simulink library "BAMLIB564xL"  (R2016b)
settings: Solver=FixedStepDiscrete  StartTime=0.0  StopTime=10.0  RelTol=1e-3  EnableMultiTasking=on
undefined symbols (not defined in the file or in its folder): Kx, Ky, ps32Table, s32A1, s32A2, s32ArgDcBusMsr, s32B0, s32B1, s32B2, s32CC1, s32CC2, s32HystOff, s32HystOn, s32IntegGain, s32LowerLim, s32LowerLimit, s32MidId, s32MidIdx, s32ModIndex, s32OutValOff, s32OutValOn, s32PropGain, s32RampDown, s32RampUp, s32ShamOffset, s32ShamOffset1, s32ShamOffset2, s32UpperLimit, ThetaAdj
undefined symbols (not defined in the file): CoefBuf, Order, s32C1, s32Kd, s32Kq, s32Lim, s32UpperLim, u16NSamples
(part 1 of 2)
settings Model: Creator=r61406  LastModifiedBy=eugkim01
settings SolverCC: PositivePriorityOrder=on  AutoInsertRateTranBlk=on
settings DataIOCC: LimitDataPoints=on  SaveFormat=Array  SignalLoggingSaveFormat=ModelDataLogs
settings OptimizationCC: ExpressionDepthLimit=2147483647  LifeSpan=1
settings DebuggingCC: UnderspecifiedInitializationDetection=Classic  MergeDetectMultiDrivingBlocksExec=none  SolverPrmCheckMsg=warning  FcnCallInpInsideContextMsg=warning  StateNameClashWarn=warning  StrictBusMsg=Warning  SFUnexpectedBacktrackingDiag=warning  SFNoUnconditionalDefaultTransitionDiag=warning  SFExecutionAtInitializationDiag=none
settings HardwareCC: ProdBitPerPointer=32  ProdBitPerSizeT=32  ProdBitPerPtrDiffT=32  ProdLargestAtomicFloat=None  ProdIntDivRoundTo=Undefined  ProdEndianess=Unspecified  ProdWordSize=32  ProdHWDeviceType=32-bit Generic
settings ModelReferenceCC: PropagateSignalLabelsOutOfModel=off
settings RTWCC: SystemTargetFile=ert.tlc  TemplateMakefile=ert_default_tmf  Description=Real-Time Workshop Embedded Coder (no auto configuration)  GenerateReport=on  IncludeHyperlinkInReport=on  LaunchReport=on  GenerateTraceInfo=on  GenerateTraceReport=on  GenerateTraceReportSl=on  GenerateTraceReportSf=on  GenerateTraceReportEml=on
settings CodeAppCC: IgnoreCustomStorageClasses=off  CustomSymbolStrType=$N$R$M  InternalIdentifier=Classic
settings ERTTargetCC: GenerateSampleERTMain=on  ERTCustomFileTemplate=example_file_process.tlc  ConvertIfToSwitch=off  SuppressUnreachableDefaultCases=off
settings ConfigComp: CovMetricSettings=dw  CovHtmlReporting=on  CovSaveCumulativeToWorkspaceVar=on  CovSaveSingleToWorkspaceVar=on  CovExternalEMLEnable=off

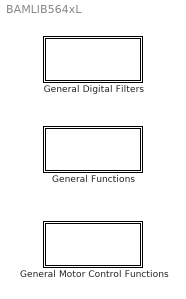
== system BAMLIB564xL ==
  General Digital Filters : Subsystem
      mask Display: disp('GDFLIB')
  General Functions : Subsystem
      mask Display: disp('GFLIB')
  General Motor Control Functions : Subsystem
      mask Display: disp('GMCLIB')

== system BAMLIB564xL/General Digital Filters ==
  GDFLIB_FilterFIR : Subsystem  mask(GDFLIB_FilterFIR){u32Order=Order, ps32CoefBuf=CoefBuf}
      mask help: The function implements FIR filter.
      mask init:
      | pos = get_param(gcb, 'Position');width = pos(3) - pos(1); height = pos(4) - pos(2);tX=width/2;tY=height*0.9;
      mask Help: web([rappid_564xl_mc_block_help,filesep,'help.html']);
      mask Display:
      | color('black');port_label('input',1,'singleIn');port_label('output',1,'singleOut');color('black');disp('GDFLIB_FilterFIR');
      | color('blue');
      | text(tX,tY, 'BAM', 'horizontalalignment', 'center');
  GDFLIB_FilterIIR1 : Subsystem  mask(GDFLIB_FilterIIR1){s32B0=s32B0, s32B1=s32B1, s32A1=s32A1}
      mask help: Bit accurate model of first order IIR filter. All parameters as well as input and output are integers.
      mask init:
      | pos = get_param(gcb, 'Position');width = pos(3) - pos(1); height = pos(4) - pos(2);tX=width/2;tY=height*0.9;
      mask Help: web([rappid_564xl_mc_block_help,filesep,'help.html']);
      mask Display: color('black');port_label('input',1,'singleIn');port_label('output',1,'singleOut');color('black');disp('GDFLIB_FilterIIR1');color('blue');text(tX,tY, 'BAM', 'horizontalAlignment', 'center');
  GDFLIB_FilterIIR2 : Subsystem  mask(GDFLIB_FilterIIR2){s32B0=s32B0, s32B1=s32B1, s32B2=s32B2, s32A1=s32A1, s32A2=s32A2}
      mask help: Bit accurate model of direct form I second order IIR filter. All parameters as well as input and output are integers.
      mask init:
      | pos = get_param(gcb, 'Position');width = pos(3) - pos(1); height = pos(4) - pos(2);tX=width/2;tY=height*0.9;
      mask Help: web([rappid_564xl_mc_block_help,filesep,'help.html']);
      mask Display: color('black');port_label('input',1,'singleIn');port_label('output',1,'singleOut');color('black');disp('GDFLIB_FilterIIR2');color('blue');text(tX,tY, 'BAM', 'horizontalAlignment', 'center');
  GDFLIB_FilterMA : Subsystem  mask(GDFLIB_FilterMA){u16NSamples=u16NSamples}
      mask help: Bit accurate model of recursive form moving average filter. All parameters as well as input and output are 32bit integers.
      mask init:
      | pos = get_param(gcb, 'Position');width = pos(3) - pos(1); height = pos(4) - pos(2);tX=width/2;tY=height*0.9;
      mask Help: web([rappid_564xl_mc_block_help,filesep,'help.html']);
      mask Display: color('black');port_label('input',1,'singleIn');port_label('output',1,'singleOut');color('black');disp('GDFLIB_FilterMA');color('blue');text(tX,tY, 'BAM', 'horizontalAlignment', 'center');

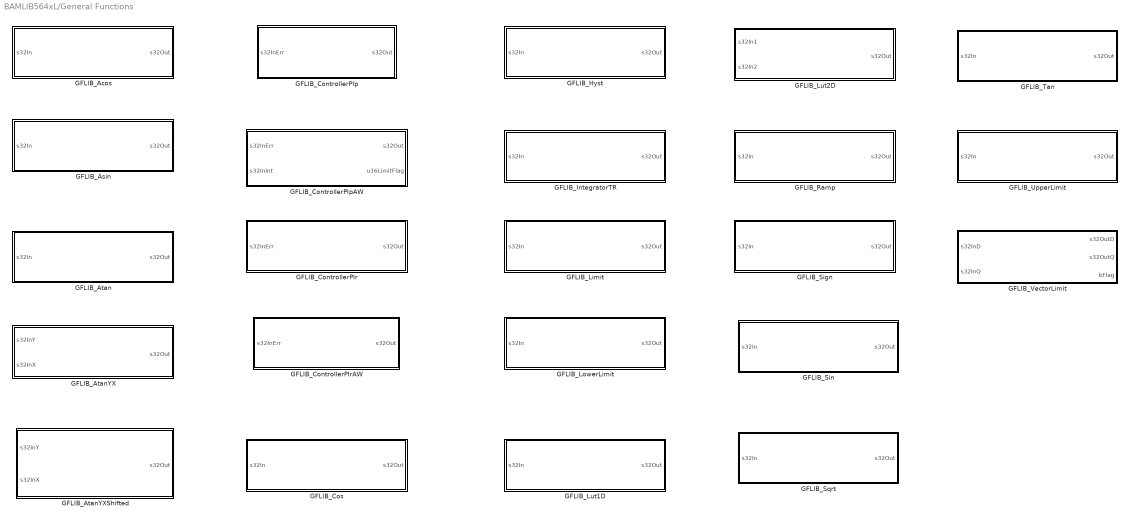
== system BAMLIB564xL/General Functions ==
  GFLIB_Acos : Subsystem  mask(GFLIB_Acos){}
      mask help: Bit accurate model of GFLIB_Acos function, which computes the acos(single) using the 4th order Taylor polynomial approximation.
      mask init:
      | pos = get_param(gcb, 'Position');width = pos(3) - pos(1); height = pos(4) - pos(2);tX=width/2;tY=height*0.9;
      mask Help: web([rappid_564xl_mc_block_help,filesep,'help.html']);
      mask Display: color('black');port_label('input',1,'singleIn');port_label('output',1,'singleOut');color('black');disp('GFLIB_Acos');color('blue');text(tX,tY, 'BAM', 'horizontalAlignment', 'center');
  GFLIB_Asin : Subsystem  mask(GFLIB_Asin){}
      mask help: Bit accurate model of GFLIB_Asin function, which computes the asin(single) using the 4th order Taylor polynomial approximation.
      mask init:
      | pos = get_param(gcb, 'Position');width = pos(3) - pos(1); height = pos(4) - pos(2);tX=width/2;tY=height*0.9;
      mask Help: web([rappid_564xl_mc_block_help,filesep,'help.html']);
      mask Display: color('black');port_label('input',1,'singleIn');port_label('output',1,'singleOut');color('black');disp('GFLIB_Asin');color('blue');text(tX,tY, 'BAM', 'horizontalAlignment', 'center');
  GFLIB_Atan : Subsystem  mask(GFLIB_Atan){}
      mask help: Bit accurate model of GFLIB_Atan function, which computes the atan(single) using the 4th order Taylor polynomial approximation.
      mask init:
      | pos = get_param(gcb, 'Position');width = pos(3) - pos(1); height = pos(4) - pos(2);tX=width/2;tY=height*0.9;
      mask Help: web([rappid_564xl_mc_block_help,filesep,'help.html']);
      mask Display: color('black');port_label('input',1,'singleIn');port_label('output',1,'singleOut');color('black');disp('GFLIB_Atan');color('blue');text(tX,tY, 'BAM', 'horizontalAlignment', 'center');
  GFLIB_AtanYX : Subsystem  mask(GFLIB_AtanYX){}
      mask help: Bit accurate model of GFLIB_AtanYX function.
      mask init:
      | pos = get_param(gcb, 'Position');width = pos(3) - pos(1); height = pos(4) - pos(2);tX=width/2;tY=height*0.9;
      mask Help: web([rappid_564xl_mc_block_help,filesep,'help.html']);
      mask Display: color('black');port_label('input',1,'singleInY');port_label('input',2,'singleInX');port_label('output',1,'singleOut');color('black');disp('GFLIB_AtanYX');color('blue');text(tX,tY, 'BAM', 'horizontalAlignment', 'center');
  GFLIB_AtanYXShifted : Subsystem  mask{Ky=Ky, Kx=Kx, ThetaAdj=ThetaAdj}
      mask help: Bit accurate model of AtanYXShifted function
      mask init:
      | pos = get_param(gcb, 'Position');width = pos(3) - pos(1); height = pos(4) - pos(2);tX=width/2;tY=height*0.9;
      mask Help: web([rappid_564xl_mc_block_help,filesep,'help.html']);
      mask Display:
      | color('black');
      | port_label('input',1, 'singleInY');
      | port_label('input',2, 'singleInX');
      | port_label('output', 1, 'singleOut');
      | color('black');
      | disp('GFLIB_AtanYXShifted');
      | color('blue');
      | text(tX,tY, 'BAM', 'horizontalAlignment', 'center');
  GFLIB_ControllerPIp : Subsystem  mask(GFLIB_ControllerPIp){s32PropGain=s32PropGain, s32IntegGain=s32IntegGain}
      mask help: Bit accurate model of parallel form PI controller without anti-windup. All parameters as well as input and output are integers.
      mask init:
      | pos = get_param(gcb, 'Position');width = pos(3) - pos(1); height = pos(4) - pos(2);tX=width/2;tY=height*0.9;
      mask Help: web([rappid_564xl_mc_block_help,filesep,'help.html']);
      mask Display: color('black');port_label('input',1,'singleInErr');port_label('output',1,'singleOut');color('black');disp('GFLIB_ControllerPIp');color('blue');text(tX,tY, 'BAM', 'horizontalAlignment', 'center');
  GFLIB_ControllerPIpAW : Subsystem  mask(GFLIB_ControllerPIpAW){s32PropGain=s32PropGain, s32IntegGain=s32IntegGain, s32UpperLimit=s32UpperLimit, s32LowerLimit=s32LowerLimit}
      mask help: Bit accurate model of parallel form PI controller with anti-windup. All parameters as well as input and output are single precision float.
      mask init:
      | pos = get_param(gcb, 'Position');width = pos(3) - pos(1); height = pos(4) - pos(2);tX=width/2;tY=height*0.9;
      mask Help: web([rappid_564xl_mc_block_help,filesep,'help.html']);
      mask Display: color('black');port_label('input',1,'singleInErr');port_label('output',1,'singleOut');port_label('output',2,'u16LimitFlag');color('black');disp('GFLIB_ControllerPIpAW');color('blue');text(tX,tY, 'BAM', 'horizontalAlignment', 'center');
  GFLIB_ControllerPIr : Subsystem  mask(GFLIB_ControllerPIr){s32CC1=s32CC1, s32CC2=s32CC2}
      mask help: Bit accurate model of reccurent form Pi controller without anti-windup. All parameters as well as input and output are single precision floating point.
      mask init:
      | pos = get_param(gcb, 'Position');width = pos(3) - pos(1); height = pos(4) - pos(2);tX=width/2;tY=height*0.9;
      mask Help: web([rappid_564xl_mc_block_help,filesep,'help.html']);
      mask Display: color('black');port_label('input',1,'singleInErr');port_label('output',1,'singleOut');color('black');disp('GFLIB_ControllerPIr');color('blue');text(tX,tY, 'BAM', 'horizontalAlignment', 'center');
  GFLIB_ControllerPIrAW : Subsystem  mask(GFLIB_ControllerPIrAW){s32CC1=s32CC1, s32CC2=s32CC2, s32UpperLimit=s32UpperLimit, s32LowerLimit=s32LowerLimit}
      mask help: Bit accurate model of reccurent form PI controller with anti-windup. All parameters as well as input and output are 32bit integers except for u16NShift parameter which is 16bit unsigned integer.
      mask init:
      | pos = get_param(gcb, 'Position');width = pos(3) - pos(1); height = pos(4) - pos(2);tX=width/2;tY=height*0.9;
      mask Help: web([rappid_564xl_mc_block_help,filesep,'help.html']);
      mask Display: color('black');port_label('input',1,'singleInErr');port_label('output',1,'singleOut');color('black');disp('GFLIB_ControllerPIrAW');color('blue');text(tX,tY, 'BAM', 'horizontalAlignment', 'center');
  GFLIB_Cos : Subsystem  mask(GFLIB_Cos){}
      mask help: Bit accurate model of GFLIB_Cos function, which computes the cos(pi * single) using the 9th order Taylor polynomial approximation.
      mask init:
      | pos = get_param(gcb, 'Position');width = pos(3) - pos(1); height = pos(4) - pos(2);tX=width/2;tY=height*0.9;
      mask Help: web([rappid_564xl_mc_block_help,filesep,'help.html']);
      mask Display: color('black');port_label('input',1,'singleIn');port_label('output',1,'singleOut');color('black');disp('GFLIB_Cos');color('blue');text(tX,tY, 'BAM', 'horizontalAlignment', 'center');
  GFLIB_Hyst : Subsystem  mask(GFLIB_Hyst){s32HystOn=s32HystOn, s32HystOff=s32HystOff, s32OutValOn=s32OutValOn, s32OutValOff=s32OutValOff}
      mask help: Bit accurate model of hysteresis function. All parameters as well as input and output are 32bit integers.
      mask init:
      | pos = get_param(gcb, 'Position');width = pos(3) - pos(1); height = pos(4) - pos(2);tX=width/2;tY=height*0.9;
      mask Help: web([rappid_564xl_mc_block_help,filesep,'help.html']);
      mask Display: color('black');port_label('input',1,'singleIn');port_label('output',1,'singleOut');color('black');disp('GFLIB_Hyst');color('blue');text(tX,tY, 'BAM', 'horizontalAlignment', 'center');
  GFLIB_IntegratorTR : Subsystem  mask(GFLIB_IntegratorTR){s32C1=s32C1}
      mask help: Bit accurate model of discrete trapezoidal integrator. All parameters as well as input and output are 32bit integers.
      mask init:
      | pos = get_param(gcb, 'Position');width = pos(3) - pos(1); height = pos(4) - pos(2);tX=width/2;tY=height*0.9;
      mask Help: web([rappid_564xl_mc_block_help,filesep,'help.html']);
      mask Display: color('black');port_label('input',1,'singleIn');port_label('output',1,'singleOut');color('black');disp('GFLIB_IntegratorTR');color('blue');text(tX,tY, 'BAM', 'horizontalAlignment', 'center');
  GFLIB_Limit : Subsystem  mask(GFLIB_Limit){s32UpperLimit=s32UpperLimit, s32LowerLim=s32LowerLim}
      mask help: Bit accurate model of GFLIB_Limit function
      mask init:
      | pos = get_param(gcb, 'Position');width = pos(3) - pos(1); height = pos(4) - pos(2);tX=width/2;tY=height*0.9;
      mask Help: web([rappid_564xl_mc_block_help,filesep,'help.html']);
      mask Display: color('black');port_label('input',1,'singleIn');port_label('output',1,'singleOut');color('black');disp('GFLIB_Limit');color('blue');text(tX,tY, 'BAM', 'horizontalAlignment', 'center');
  GFLIB_LowerLimit : Subsystem  mask(GFLIB_LowerLimit){s32LowerLim=s32LowerLim}
      mask help: Bit accurate model of GFLIB_LowerLimit function
      mask init:
      | pos = get_param(gcb, 'Position');width = pos(3) - pos(1); height = pos(4) - pos(2);tX=width/2;tY=height*0.9;
      mask Help: web([rappid_564xl_mc_block_help,filesep,'help.html']);
      mask Display: color('black');port_label('input',1,'singleIn');port_label('output',1,'singleOut');color('black');disp('GFLIB_LowerLimit');color('blue');text(tX,tY, 'BAM', 'horizontalAlignment', 'center');
  GFLIB_Lut1D : Subsystem  mask(GFLIB_Lut1D){s32ShamOffset=s32ShamOffset, ps32Table=ps32Table, s32MidIdx=s32MidIdx}
      mask help: Bit accurate model of GFLIB_Lut1D function
      mask init:
      | pos = get_param(gcb, 'Position');width = pos(3) - pos(1); height = pos(4) - pos(2);tX=width/2;tY=height*0.9;
      mask Help: web([rappid_564xl_mc_block_help,filesep,'help.html']);
      mask Display: color('black');port_label('input',1,'singleIn');port_label('output',1,'singleOut');color('black');disp('GFLIB_Lut1D');color('blue');text(tX,tY, 'BAM', 'horizontalAlignment', 'center');
  GFLIB_Lut2D : Subsystem  mask(GFLIB_Lut2D){s32ShamOffset1=s32ShamOffset1, s32ShamOffset2=s32ShamOffset2, ps32Table=ps32Table, s32MidId=s32MidId}
      mask help: Bit accurate model of GFLIB_Lut2D function
      mask init:
      | pos = get_param(gcb, 'Position');width = pos(3) - pos(1); height = pos(4) - pos(2);tX=width/2;tY=height*0.9;
      mask Help: web([rappid_564xl_mc_block_help,filesep,'help.html']);
      mask Display: color('black');port_label('input',1,'singleIn1');port_label('input',2,'singleIn2');port_label('output',1,'singleOut');color('black');disp('GFLIB_Lut2D');color('blue');text(tX,tY, 'BAM', 'horizontalAlignment', 'center');
  GFLIB_Ramp : Subsystem  mask(GFLIB_Ramp){s32RampUp=s32RampUp, s32RampDown=s32RampDown}
      mask help: Bit accurate model of ramp function. All parameters as well as input and output are 32bit integers.
      mask init:
      | pos = get_param(gcb, 'Position');width = pos(3) - pos(1); height = pos(4) - pos(2);tX=width/2;tY=height*0.9;
      mask Help: web([rappid_564xl_mc_block_help,filesep,'help.html']);
      mask Display: color('black');port_label('input',1,'singleIn');port_label('output',1,'singleOut');color('black');disp('GFLIB_Ramp');color('blue');text(tX,tY, 'BAM', 'horizontalAlignment', 'center');
  GFLIB_Sign : Subsystem  mask(GFLIB_Sign){}
      mask help: Bit accurate model of Sign function
      mask init:
      | pos = get_param(gcb, 'Position');width = pos(3) - pos(1); height = pos(4) - pos(2);tX=width/2;tY=height*0.9;
      mask Help: web([rappid_564xl_mc_block_help,filesep,'help.html']);
      mask Display: color('black');port_label('input',1,'singleIn');port_label('output',1,'singleOut');color('black');disp('GFLIB_Sign');color('blue');text(tX,tY, 'BAM', 'horizontalAlignment', 'center');
  GFLIB_Sin : Subsystem  mask(GFLIB_Sin){}
      mask help: Bit accurate model of GFLIB_Sin function, which computes the sin(pi * single) using the 9th order Taylor polynomial approximation.
      mask init:
      | pos = get_param(gcb, 'Position');width = pos(3) - pos(1); height = pos(4) - pos(2);tX=width/2;tY=height*0.9;
      mask Help: web([rappid_564xl_mc_block_help,filesep,'help.html']);
      mask Display: color('black');port_label('input',1,'singleIn');port_label('output',1,'singleOut');color('black');disp('GFLIB_Sin');color('blue');text(tX,tY, 'BAM', 'horizontalAlignment', 'center');
  GFLIB_Sqrt : Subsystem  mask(GFLIB_Sqrt){}
      mask help: Bit accurate model of GFLIB_Sqrt function, which computes the square root of input argument using the Newton-Raphson iterations preceeded by normalization and tentative approximation.
      mask init:
      | pos = get_param(gcb, 'Position');width = pos(3) - pos(1); height = pos(4) - pos(2);tX=width/2;tY=height*0.9;
      mask Help: web([rappid_564xl_mc_block_help,filesep,'help.html']);
      mask Display: color('black');port_label('input',1,'singleIn');port_label('output',1,'singleOut');color('black');disp('GFLIB_Sqrt');color('blue');text(tX,tY, 'BAM', 'horizontalAlignment', 'center');
  GFLIB_Tan : Subsystem  mask(GFLIB_Tan){}
      mask help: Bit accurate model of GFLIB_Tan function, which computes the tan(pi * single) using the 4th order Taylor polynomial approximation.
      mask init:
      | pos = get_param(gcb, 'Position');width = pos(3) - pos(1); height = pos(4) - pos(2);tX=width/2;tY=height*0.9;
      mask Help: web([rappid_564xl_mc_block_help,filesep,'help.html']);
      mask Display: color('black');port_label('input',1,'singleIn');port_label('output',1,'singleOut');color('black');disp('GFLIB_Tan');color('blue');text(tX,tY, 'BAM', 'horizontalAlignment', 'center');
  GFLIB_UpperLimit : Subsystem  mask(GFLIB_UpperLimit){s32UpperLim=s32UpperLim}
      mask help: Bit accurate model of GFLIB_UpperLimit function
      mask init:
      | pos = get_param(gcb, 'Position');width = pos(3) - pos(1); height = pos(4) - pos(2);tX=width/2;tY=height*0.9;
      mask Help: web([rappid_564xl_mc_block_help,filesep,'help.html']);
      mask Display: color('black');port_label('input',1,'singleIn');port_label('output',1,'singleOut');color('black');disp('GFLIB_UpperLimit');color('blue');text(tX,tY, 'BAM', 'horizontalAlignment', 'center');
  GFLIB_VectorLimit : Subsystem  mask(GFLIB_VectorLimit){s32Lim=s32Lim}
      mask help: Bit accurate model of GFLIB_VectorLimit function
      mask init:
      | pos = get_param(gcb, 'Position');width = pos(3) - pos(1); height = pos(4) - pos(2);tX=width/2;tY=height*0.9;
      mask Help: web([rappid_564xl_mc_block_help,filesep,'help.html']);
      mask Display: color('black');port_label('input',1,'singleInD');port_label('input',2,'singleInQ');port_label('output',1,'singleOutD');port_label('output',2,'singleOutQ');port_label('output',3,'bFlag');color('black');disp('GFLIB_VectorLimit');color('blue');text(tX,tY, 'BAM', 'horizontalAlignment', 'center');

== system BAMLIB564xL/General Motor Control Functions ==
  GMCLIB_Clark : Subsystem  mask(GMCLIB_Clark){}
      mask help: Bit accurate model of Clarke transformation 3ph -> 2ph
      mask init:
      | pos = get_param(gcb, 'Position');width = pos(3) - pos(1); height = pos(4) - pos(2);tX=width/2;tY=height*0.9;
      mask Help: web([rappid_564xl_mc_block_help,filesep,'help.html']);
      mask Display: color('black');port_label('input',1,'singleA');port_label('input',2,'singleB');port_label('input',3,'singleC');port_label('output',1,'singleAlpha');port_label('output',2,'singleBeta');color('black');disp('GMCLIB_Clark');color('blue');text(tX,tY, 'BAM', 'horizontalAlignment', 'center');
  GMCLIB_ClarkInv : Subsystem  mask(GMCLIB_ClarkInv){}
      mask help: Bit accurate model of inverse Clarke transformation 2ph -> 3ph
      mask init:
      | pos = get_param(gcb, 'Position');width = pos(3) - pos(1); height = pos(4) - pos(2);tX=width/2;tY=height*0.9;
      mask Help: web([rappid_564xl_mc_block_help,filesep,'help.html']);
      mask Display: color('black');port_label('input',1,'singleAlpha');port_label('input',2,'singleBeta');port_label('output',1,'singleA');port_label('output',2,'singleB');port_label('output',3,'singleC');color('black');disp('GMCLIB_ClarkInv');color('blue');text(tX,tY, 'BAM', 'horizontalAlignment', 'center');
  GMCLIB_DecouplingPMSM : Subsystem  mask(GMCLIB_DecouplingPMSM){s32Ld=s32Kd, s32Lq=s32Kq}
      mask help: Bit accurate model of decoupling for PMSM model
      mask init:
      | pos = get_param(gcb, 'Position');width = pos(3) - pos(1); height = pos(4) - pos(2);tX=width/2;tY=height*0.9;
      mask Help: web([rappid_564xl_mc_block_help,filesep,'help.html']);
      mask Display: color('black');port_label('input',1,'singleUd');port_label('input',2,'singleUq');port_label('input',3,'singleId');port_label('input',4,'singleIq');port_label('input',5,'singleAngVel');port_label('output',1,'singleUdDec');port_label('output',2,'singleUqDec');color('black');disp('GMCLIB_DecouplingPMSM');color('blue');text(tX,tY, 'BAM', 'horizontalAlignment', 'center');
  GMCLIB_ElimDcBusRip : Subsystem  mask(GMCLIB_ElimDcBusRip){s32ModIndex=s32ModIndex, s32ArgDcBusMsr=s32ArgDcBusMsr}
      mask help: Bit accurate model of DC Bus voltage ripple elimination function
      mask init:
      | pos = get_param(gcb, 'Position');width = pos(3) - pos(1); height = pos(4) - pos(2);tX=width/2;tY=height*0.9;
      mask Help: web([rappid_564xl_mc_block_help,filesep,'help.html']);
      mask Display: color('black');port_label('input',1,'singleAlpha');port_label('input',2,'singleBeta');port_label('output',1,'singleAlphaOut');port_label('output',2,'singleBetaOut');color('black');disp('GMCLIB_ElimDcBusRip');color('blue');text(tX,tY, 'BAM', 'horizontalAlignment', 'center');
  GMCLIB_Park : Subsystem  mask(GMCLIB_Park){}
      mask help: Bit accurate model of Park transformation 2ph stationary -> 2ph rotational
      mask init:
      | pos = get_param(gcb, 'Position');width = pos(3) - pos(1); height = pos(4) - pos(2);tX=width/2;tY=height*0.9;
      mask Help: web([rappid_564xl_mc_block_help,filesep,'help.html']);
      mask Display: color('black');port_label('input',1,'singleAlpha');port_label('input',2,'singleBeta');port_label('input',3,'singleSin');port_label('input',4,'singleCos');port_label('output',1,'singleD');port_label('output',2,'singleQ');color('black');disp('GMCLIB_Park');color('blue');text(tX,tY, 'BAM', 'horizontalAlignment', 'center');
  GMCLIB_ParkInv : Subsystem  mask(GMCLIB_ParkInv){}
      mask help: Bit accurate model of Inverse Park transformation 2ph rotational -> 2ph stationary
      mask init:
      | pos = get_param(gcb, 'Position');width = pos(3) - pos(1); height = pos(4) - pos(2);tX=width/2;tY=height*0.9;
      mask Help: web([rappid_564xl_mc_block_help,filesep,'help.html']);
      mask Display: color('black');port_label('input',1,'singleD');port_label('input',2,'singleQ');port_label('input',3,'singleSin');port_label('input',4,'singleCos');port_label('output',1,'singleAlpha');port_label('output',2,'singleBeta');color('black');disp('GMCLIB_ParkInv');color('blue');text(tX,tY, 'BAM', 'horizontalAlignment', 'center');
  GMCLIB_SvmStd : Subsystem  mask(GMCLIB_SvmStd){}
      mask help: Bit accurate model of Standard Space Vector Modulation
      mask init:
      | pos = get_param(gcb, 'Position');width = pos(3) - pos(1); height = pos(4) - pos(2);tX=width/2;tY=height*0.9;
      mask Help: web([rappid_564xl_mc_block_help,filesep,'help.html']);
      mask Display: color('black');port_label('input',1,'singleIn1');port_label('input',2,'singleIn2');port_label('output',1,'singleOut1');port_label('output',2,'singleOut2');port_label('output',3,'singleOut3');port_label('output',4,'singleSector');color('black');disp('GMCLIB_SvmStd');color('blue');text(tX,tY, 'BAM', 'horizontalAlignment', 'center');

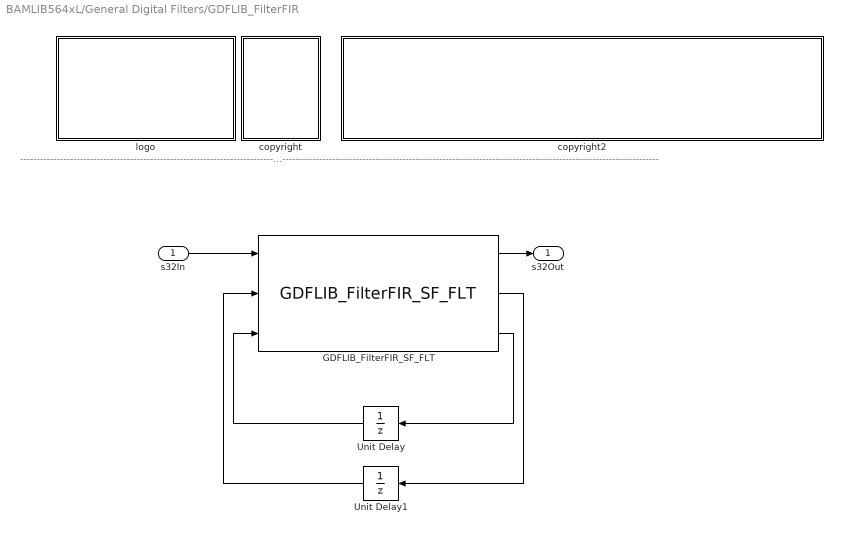
== system BAMLIB564xL/General Digital Filters/GDFLIB_FilterFIR ==
  note: ---------------------------------------------------------------------------------------------------------------------------------------------------------------------------------------------------
  s32In : Inport
  GDFLIB_FilterFIR_SF_FLT : S-Function  FunctionName=GDFLIB_FilterFIR_SF_FLT  Parameters=u32Order, ps32CoefBuf  SFunctionDeploymentMode=off  EnableBusSupport=off
  Unit Delay : UnitDelay  SampleTime=-1
  Unit Delay1 : UnitDelay  SampleTime=-1
  copyright : Subsystem
      mask Display: text(10,90,'FILE:');text(10,75,'DESRIPTION:')text(10,60,'COPYRIGHT:')text(10,45,'VERSION:')text(10,30,'DATE:')text(10,15,'AUTHOR:')
  copyright2 : Subsystem
      mask Display: text(10,90,'GDFLIB_FilterFIR_BAM_FLT.mdl');text(10,75,'FilterFIR transformation');text(10,60,'Freescale')text(10,45,'0.1');text(10,30,'29-Sep-2010');text(10,15,'');
  logo : Subsystem
      mask Display: image(imread('logo.jpg'))
  s32Out : Outport
  wires:
  Unit Delay1/1 -> GDFLIB_FilterFIR_SF_FLT/2
  Unit Delay/1 -> GDFLIB_FilterFIR_SF_FLT/3
  GDFLIB_FilterFIR_SF_FLT/2 -> Unit Delay1/1
  GDFLIB_FilterFIR_SF_FLT/3 -> Unit Delay/1
  GDFLIB_FilterFIR_SF_FLT/1 -> s32Out/1
  s32In/1 -> GDFLIB_FilterFIR_SF_FLT/1

== system BAMLIB564xL/General Digital Filters/GDFLIB_FilterIIR1 ==
  note: ---------------------------------------------------------------------------------------------------------------------------------------------------------------------------------------------------
  s32In : Inport
  GDFLIB_FilterIIR1_SF_FLT : S-Function  FunctionName=GDFLIB_FilterIIR1_SF_FLT  Parameters=s32B0,s32B1,s32A1  SFunctionDeploymentMode=off  EnableBusSupport=off
  Unit Delay : UnitDelay  SampleTime=-1
  Unit Delay1 : UnitDelay  SampleTime=-1
  copyright : Subsystem
      mask Display: text(10,90,'FILE:');text(10,75,'DESRIPTION:')text(10,60,'COPYRIGHT:')text(10,45,'VERSION:')text(10,30,'DATE:')text(10,15,'AUTHOR:')
  copyright2 : Subsystem
      mask Display: text(10,90,'GDFLIB_FilterIIR1_BAM_FLT.mdl');text(10,75,'Direct form I first order IIR filter.');text(10,60,'Freescale')text(10,45,'0.1');text(10,30,'29-Sep-2010');text(10,15,'');
  logo : Subsystem
      mask Display: image(imread('logo.jpg'))
  s32Out : Outport
  wires:
  Unit Delay1/1 -> GDFLIB_FilterIIR1_SF_FLT/2
  Unit Delay/1 -> GDFLIB_FilterIIR1_SF_FLT/3
  GDFLIB_FilterIIR1_SF_FLT/3 -> Unit Delay/1
  GDFLIB_FilterIIR1_SF_FLT/2 -> Unit Delay1/1
  GDFLIB_FilterIIR1_SF_FLT/1 -> s32Out/1
  s32In/1 -> GDFLIB_FilterIIR1_SF_FLT/1

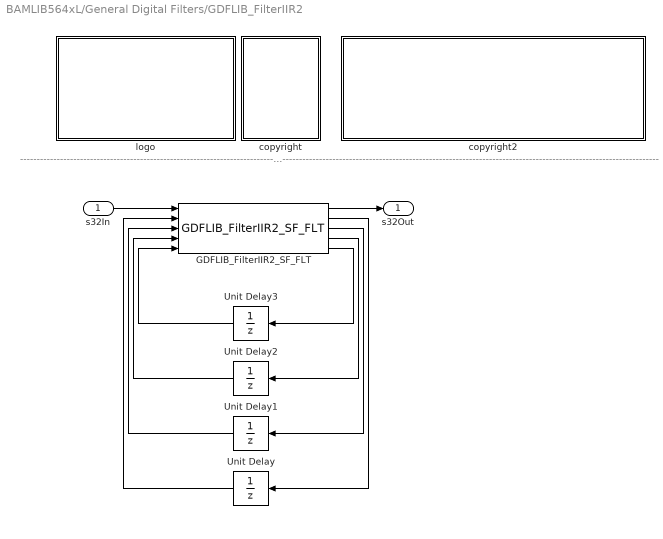
== system BAMLIB564xL/General Digital Filters/GDFLIB_FilterIIR2 ==
  note: ---------------------------------------------------------------------------------------------------------------------------------------------------------------------------------------------------
  s32In : Inport
  GDFLIB_FilterIIR2_SF_FLT : S-Function  FunctionName=GDFLIB_FilterIIR2_SF_FLT  Parameters=s32B0,s32B1,s32B2,s32A1,s32A2  SFunctionDeploymentMode=off  EnableBusSupport=off
  Unit Delay{,1..3} (4 alike) : UnitDelay  SampleTime=-1
  copyright : Subsystem
      mask Display: text(10,90,'FILE:');text(10,75,'DESRIPTION:')text(10,60,'COPYRIGHT:')text(10,45,'VERSION:')text(10,30,'DATE:')text(10,15,'AUTHOR:')
  copyright2 : Subsystem
      mask Display: text(10,90,'GDFLIB_FilterIIR2_BAM_FLT.mdl');text(10,75,'Direct form I second order IIR filter.');text(10,60,'Freescale')text(10,45,'0.1');text(10,30,'29-Sep-2010');text(10,15,'');
  logo : Subsystem
      mask Display: image(imread('logo.jpg'))
  s32Out : Outport
  wires:
  Unit Delay3/1 -> GDFLIB_FilterIIR2_SF_FLT/5
  GDFLIB_FilterIIR2_SF_FLT/5 -> Unit Delay3/1
  Unit Delay2/1 -> GDFLIB_FilterIIR2_SF_FLT/4
  GDFLIB_FilterIIR2_SF_FLT/4 -> Unit Delay2/1
  Unit Delay1/1 -> GDFLIB_FilterIIR2_SF_FLT/3
  GDFLIB_FilterIIR2_SF_FLT/3 -> Unit Delay1/1
  Unit Delay/1 -> GDFLIB_FilterIIR2_SF_FLT/2
  GDFLIB_FilterIIR2_SF_FLT/2 -> Unit Delay/1
  GDFLIB_FilterIIR2_SF_FLT/1 -> s32Out/1
  s32In/1 -> GDFLIB_FilterIIR2_SF_FLT/1

== system BAMLIB564xL/General Digital Filters/GDFLIB_FilterMA ==
  note: ---------------------------------------------------------------------------------------------------------------------------------------------------------------------------------------------------
  s32In : Inport
  GDFLIB_FilterMA_SF_FLT : S-Function  FunctionName=GDFLIB_FilterMA_SF_FLT  Parameters=u16NSamples  SFunctionDeploymentMode=off  EnableBusSupport=off
  Unit Delay : UnitDelay  SampleTime=-1
  copyright : Subsystem
      mask Display: text(10,90,'FILE:');text(10,75,'DESRIPTION:')text(10,60,'COPYRIGHT:')text(10,45,'VERSION:')text(10,30,'DATE:')text(10,15,'AUTHOR:')
  copyright2 : Subsystem
      mask Display: text(10,90,'GDFLIB_FilterMA_BAM_FLT.mdl');text(10,75,'Recursive form moving average filter.');text(10,60,'Freescale')text(10,45,'0.1');text(10,30,'29-Sep-2010');text(10,15,'');
  logo : Subsystem
      mask Display: image(imread('logo.jpg'))
  s32Out : Outport
  wires:
  Unit Delay/1 -> GDFLIB_FilterMA_SF_FLT/2
  GDFLIB_FilterMA_SF_FLT/2 -> Unit Delay/1
  GDFLIB_FilterMA_SF_FLT/1 -> s32Out/1
  s32In/1 -> GDFLIB_FilterMA_SF_FLT/1

== system BAMLIB564xL/General Functions/GFLIB_Acos ==
  note: ---------------------------------------------------------------------------------------------------------------------------------------------------------------------------------------------------
  s32In : Inport
  GFLIB_Acos_SF_FLT : S-Function  FunctionName=GFLIB_Acos_SF_FLT  SFunctionDeploymentMode=off  EnableBusSupport=off
  copyright : Subsystem
      mask Display: text(10,90,'FILE:');text(10,75,'DESRIPTION:')text(10,60,'COPYRIGHT:')text(10,45,'VERSION:')text(10,30,'DATE:')text(10,15,'AUTHOR:')
  copyright2 : Subsystem
      mask Display: text(10,90,'GFLIB_Acos_BAM_FLT.mdl');text(10,75,'Inverse cosine transformation');text(10,60,'Freescale')text(10,45,'0.1');text(10,30,'29-Sep-2010');text(10,15,'');
  logo : Subsystem
      mask Display: image(imread('logo.jpg'))
  s32Out : Outport
  wires:
  GFLIB_Acos_SF_FLT/1 -> s32Out/1
  s32In/1 -> GFLIB_Acos_SF_FLT/1

== system BAMLIB564xL/General Functions/GFLIB_Asin ==
  note: ---------------------------------------------------------------------------------------------------------------------------------------------------------------------------------------------------
  s32In : Inport
  GFLIB_Asin_SF_FLT : S-Function  FunctionName=GFLIB_Asin_SF_FLT  SFunctionDeploymentMode=off  EnableBusSupport=off
  copyright : Subsystem
      mask Display: text(10,90,'FILE:');text(10,75,'DESRIPTION:')text(10,60,'COPYRIGHT:')text(10,45,'VERSION:')text(10,30,'DATE:')text(10,15,'AUTHOR:')
  copyright2 : Subsystem
      mask Display: text(10,90,'GFLIB_Asin_BAM_FLT.mdl');text(10,75,'ArcSine of argument.');text(10,60,'Freescale')text(10,45,'0.1');text(10,30,'29-Sep-2010');text(10,15,'');
  logo : Subsystem
      mask Display: image(imread('logo.jpg'))
  s32Out : Outport
  wires:
  GFLIB_Asin_SF_FLT/1 -> s32Out/1
  s32In/1 -> GFLIB_Asin_SF_FLT/1

== system BAMLIB564xL/General Functions/GFLIB_Atan ==
  note: ---------------------------------------------------------------------------------------------------------------------------------------------------------------------------------------------------
  s32In : Inport
  GFLIB_Atan_SF_FLT : S-Function  FunctionName=GFLIB_Atan_SF_FLT  SFunctionDeploymentMode=off  EnableBusSupport=off
  copyright : Subsystem
      mask Display: text(10,90,'FILE:');text(10,75,'DESRIPTION:')text(10,60,'COPYRIGHT:')text(10,45,'VERSION:')text(10,30,'DATE:')text(10,15,'AUTHOR:')
  copyright2 : Subsystem
      mask Display: text(10,90,'GFLIB_Atan_BAM_FLT.mdl');text(10,75,'Arctangent of argument.');text(10,60,'Freescale')text(10,45,'0.1');text(10,30,'29-Sep-2010');text(10,15,'');
  logo : Subsystem
      mask Display: image(imread('logo.jpg'))
  s32Out : Outport
  wires:
  GFLIB_Atan_SF_FLT/1 -> s32Out/1
  s32In/1 -> GFLIB_Atan_SF_FLT/1

== system BAMLIB564xL/General Functions/GFLIB_AtanYX ==
  note: ---------------------------------------------------------------------------------------------------------------------------------------------------------------------------------------------------
  s32InY : Inport
  s32InX : Inport  Port=2
  GFLIB_AtanYX_SF_FLT : S-Function  FunctionName=GFLIB_AtanYX_SF_FLT  SFunctionDeploymentMode=off  EnableBusSupport=off
  copyright : Subsystem
      mask Display: text(10,90,'FILE:');text(10,75,'DESRIPTION:')text(10,60,'COPYRIGHT:')text(10,45,'VERSION:')text(10,30,'DATE:')text(10,15,'AUTHOR:')
  copyright2 : Subsystem
      mask Display: text(10,90,'GFLIB_AtanYX_BAM_FLT.mdl');text(10,75,'YX Arctangent of argument.');text(10,60,'Freescale')text(10,45,'0.1');text(10,30,'29-Sep-2010');text(10,15,'');
  logo : Subsystem
      mask Display: image(imread('logo.jpg'))
  s32Out : Outport
  wires:
  GFLIB_AtanYX_SF_FLT/1 -> s32Out/1
  s32InX/1 -> GFLIB_AtanYX_SF_FLT/2
  s32InY/1 -> GFLIB_AtanYX_SF_FLT/1

== system BAMLIB564xL/General Functions/GFLIB_AtanYXShifted ==
  note: ---------------------------------------------------------------------------------------------------------------------------------------------------------------------------------------------------
  s32InY : Inport
  s32InX : Inport  Port=2
  GFLIB_AtanYXShifted_SF_FLT : S-Function  FunctionName=GFLIB_AtanYXShifted_SF_FLT  Parameters=Ky,Kx,ThetaAdj  SFunctionDeploymentMode=off  EnableBusSupport=off
  copyright : Subsystem
      mask Display: text(10,90,'FILE:');text(10,75,'DESRIPTION:')text(10,60,'COPYRIGHT:')text(10,45,'VERSION:')text(10,30,'DATE:')text(10,15,'AUTHOR:')
  copyright2 : Subsystem
      mask Display:
      | text(10,90,'GFLIB_AtanYXShifted_BAM_FLT.mdl');
      | text(10,75,'AtanYXShifted function');
      | text(10,60,'Freescale & ST Microelectronics');
      | text(10,45,'0.1');
      | text(10,30,'31-Nov-2009');
      | text(10,15,'Andrzej Lara');
  logo : Subsystem
      mask Display: image(imread('logo.jpg'))
  s32Out : Outport
  wires:
  GFLIB_AtanYXShifted_SF_FLT/1 -> s32Out/1
  s32InX/1 -> GFLIB_AtanYXShifted_SF_FLT/2
  s32InY/1 -> GFLIB_AtanYXShifted_SF_FLT/1

== system BAMLIB564xL/General Functions/GFLIB_ControllerPIp ==
  note: ---------------------------------------------------------------------------------------------------------------------------------------------------------------------------------------------------
  s32InErr : Inport
  GFLIB_ControllerPIp_SF_FLT : S-Function  FunctionName=GFLIB_ControllerPIp_SF_FLT  Parameters=s32PropGain,s32IntegGain  SFunctionDeploymentMode=off  EnableBusSupport=off
  Unit Delay : UnitDelay  SampleTime=-1
  Unit Delay1 : UnitDelay  SampleTime=-1
  copyright : Subsystem
      mask Display: text(10,90,'FILE:');text(10,75,'DESRIPTION:')text(10,60,'COPYRIGHT:')text(10,45,'VERSION:')text(10,30,'DATE:')text(10,15,'AUTHOR:')
  copyright2 : Subsystem
      mask Display: text(10,90,'GFLIB_ControllerPIp_BAM_FLT.mdl');text(10,75,'Parallel form of a standard PI controller without anti-windup but with saturation at maximal values of 32bit number <-2^31;2^31).');text(10,60,'Freescale')text(10,45,'0.1');text(10,30,'29-Sep-2010');text(10,15,'');
  logo : Subsystem
      mask Display: image(imread('logo.jpg'))
  s32Out : Outport
  wires:
  Unit Delay1/1 -> GFLIB_ControllerPIp_SF_FLT/2
  Unit Delay/1 -> GFLIB_ControllerPIp_SF_FLT/3
  GFLIB_ControllerPIp_SF_FLT/3 -> Unit Delay/1
  GFLIB_ControllerPIp_SF_FLT/2 -> Unit Delay1/1
  GFLIB_ControllerPIp_SF_FLT/1 -> s32Out/1
  s32InErr/1 -> GFLIB_ControllerPIp_SF_FLT/1

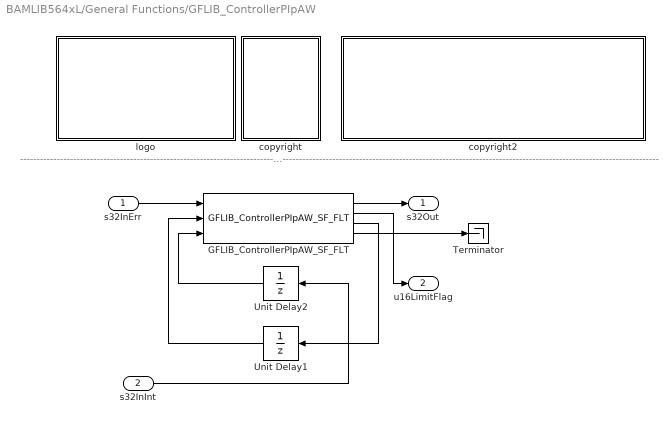
== system BAMLIB564xL/General Functions/GFLIB_ControllerPIpAW ==
  note: ---------------------------------------------------------------------------------------------------------------------------------------------------------------------------------------------------
  s32InErr : Inport
  s32InInt : Inport  Port=2
  GFLIB_ControllerPIpAW_SF_FLT : S-Function  FunctionName=GFLIB_ControllerPIpAW_SF_FLT  Parameters=s32PropGain,s32IntegGain,s32UpperLimit,s32LowerLimit  SFunctionDeploymentMode=off  EnableBusSupport=off
  Terminator : Terminator
  Unit Delay1 : UnitDelay  SampleTime=-1
  Unit Delay2 : UnitDelay  SampleTime=-1
  copyright : Subsystem
      mask Display: text(10,90,'FILE:');text(10,75,'DESRIPTION:')text(10,60,'COPYRIGHT:')text(10,45,'VERSION:')text(10,30,'DATE:')text(10,15,'AUTHOR:')
  copyright2 : Subsystem
      mask Display: text(10,90,'GFLIB_ControllerPIpAW_BAM_FLT.mdl');text(10,75,'Parallel form of a standard PI controller with implemented anti-windup.');text(10,60,'Freescale')text(10,45,'0.1');text(10,30,'31-Jan-2011');text(10,15,'');
  logo : Subsystem
      mask Display: image(imread('logo.jpg'))
  s32Out : Outport
  u16LimitFlag : Outport  Port=2
  wires:
  GFLIB_ControllerPIpAW_SF_FLT/4 -> Terminator/1
  s32InInt/1 -> Unit Delay2/1
  Unit Delay2/1 -> GFLIB_ControllerPIpAW_SF_FLT/3
  GFLIB_ControllerPIpAW_SF_FLT/2 -> u16LimitFlag/1
  Unit Delay1/1 -> GFLIB_ControllerPIpAW_SF_FLT/2
  GFLIB_ControllerPIpAW_SF_FLT/3 -> Unit Delay1/1
  GFLIB_ControllerPIpAW_SF_FLT/1 -> s32Out/1
  s32InErr/1 -> GFLIB_ControllerPIpAW_SF_FLT/1

== system BAMLIB564xL/General Functions/GFLIB_ControllerPIr ==
  note: ---------------------------------------------------------------------------------------------------------------------------------------------------------------------------------------------------
  s32InErr : Inport
  GFLIB_ControllerPIr_SF_FLT : S-Function  FunctionName=GFLIB_ControllerPIr_SF_FLT  Parameters=s32CC1,s32CC2  SFunctionDeploymentMode=off  EnableBusSupport=off
  Unit Delay : UnitDelay  SampleTime=-1
  Unit Delay1 : UnitDelay  SampleTime=-1
  copyright : Subsystem
      mask Display: text(10,90,'FILE:');text(10,75,'DESRIPTION:')text(10,60,'COPYRIGHT:')text(10,45,'VERSION:')text(10,30,'DATE:')text(10,15,'AUTHOR:')
  copyright2 : Subsystem
      mask Display: text(10,90,'GFLIB_ControllerPIr_BAM_FLT.mdl');text(10,75,'Recurrent form of a standard PI controller without anti-windup.');text(10,60,'Freescale')text(10,45,'0.1');text(10,30,'29-Sep-2010');text(10,15,'');
  logo : Subsystem
      mask Display: image(imread('logo.jpg'))
  s32Out : Outport
  wires:
  Unit Delay1/1 -> GFLIB_ControllerPIr_SF_FLT/2
  Unit Delay/1 -> GFLIB_ControllerPIr_SF_FLT/3
  GFLIB_ControllerPIr_SF_FLT/2 -> Unit Delay1/1
  GFLIB_ControllerPIr_SF_FLT/3 -> Unit Delay/1
  GFLIB_ControllerPIr_SF_FLT/1 -> s32Out/1
  s32InErr/1 -> GFLIB_ControllerPIr_SF_FLT/1

== system BAMLIB564xL/General Functions/GFLIB_ControllerPIrAW ==
  note: ---------------------------------------------------------------------------------------------------------------------------------------------------------------------------------------------------
  s32InErr : Inport
  GFLIB_ControllerPIrAW_SF_FLT : S-Function  FunctionName=GFLIB_ControllerPIrAW_SF_FLT  Parameters=s32CC1,s32CC2,s32UpperLimit,s32LowerLimit  SFunctionDeploymentMode=off  EnableBusSupport=off
  Unit Delay : UnitDelay  SampleTime=-1
  Unit Delay1 : UnitDelay  SampleTime=-1
  copyright : Subsystem
      mask Display: text(10,90,'FILE:');text(10,75,'DESRIPTION:')text(10,60,'COPYRIGHT:')text(10,45,'VERSION:')text(10,30,'DATE:')text(10,15,'AUTHOR:')
  copyright2 : Subsystem
      mask Display: text(10,90,'GFLIB_ControllerPIrAW_BAM_FLT.mdl');text(10,75,'Recurrent form of a standard PI controller with anti-windup functionality.');text(10,60,'Freescale')text(10,45,'0.1');text(10,30,'29-Sep-2010');text(10,15,'');
  logo : Subsystem
      mask Display: image(imread('logo.jpg'))
  s32Out : Outport
  wires:
  Unit Delay1/1 -> GFLIB_ControllerPIrAW_SF_FLT/2
  Unit Delay/1 -> GFLIB_ControllerPIrAW_SF_FLT/3
  GFLIB_ControllerPIrAW_SF_FLT/2 -> Unit Delay1/1
  GFLIB_ControllerPIrAW_SF_FLT/3 -> Unit Delay/1
  GFLIB_ControllerPIrAW_SF_FLT/1 -> s32Out/1
  s32InErr/1 -> GFLIB_ControllerPIrAW_SF_FLT/1

== system BAMLIB564xL/General Functions/GFLIB_Cos ==
  note: ---------------------------------------------------------------------------------------------------------------------------------------------------------------------------------------------------
  s32In : Inport
  GFLIB_Cos_SF_FLT : S-Function  FunctionName=GFLIB_Cos_SF_FLT  SFunctionDeploymentMode=off  EnableBusSupport=off
  copyright : Subsystem
      mask Display: text(10,90,'FILE:');text(10,75,'DESRIPTION:')text(10,60,'COPYRIGHT:')text(10,45,'VERSION:')text(10,30,'DATE:')text(10,15,'AUTHOR:')
  copyright2 : Subsystem
      mask Display: text(10,90,'GFLIB_Cos_BAM_FLT.mdl');text(10,75,'Cosine of argument.');text(10,60,'Freescale')text(10,45,'0.1');text(10,30,'29-Sep-2010');text(10,15,'');
  logo : Subsystem
      mask Display: image(imread('logo.jpg'))
  s32Out : Outport
  wires:
  GFLIB_Cos_SF_FLT/1 -> s32Out/1
  s32In/1 -> GFLIB_Cos_SF_FLT/1

== system BAMLIB564xL/General Functions/GFLIB_Hyst ==
  note: ---------------------------------------------------------------------------------------------------------------------------------------------------------------------------------------------------
  s32In : Inport
  GFLIB_Hyst_SF_FLT : S-Function  FunctionName=GFLIB_Hyst_SF_FLT  Parameters=s32HystOn,s32HystOff,s32OutValOn,s32OutValOff  SFunctionDeploymentMode=off  EnableBusSupport=off
  Unit Delay : UnitDelay  SampleTime=-1
  copyright : Subsystem
      mask Display: text(10,90,'FILE:');text(10,75,'DESRIPTION:')text(10,60,'COPYRIGHT:')text(10,45,'VERSION:')text(10,30,'DATE:')text(10,15,'AUTHOR:')
  copyright2 : Subsystem
      mask Display: text(10,90,'GFLIB_Hyst_BAM_FLT.mdl');text(10,75,'Hysteresis function.');text(10,60,'Freescale')text(10,45,'0.1');text(10,30,'29-Sep-2010');text(10,15,'');
  logo : Subsystem
      mask Display: image(imread('logo.jpg'))
  s32Out : Outport
  wires:
  Unit Delay/1 -> GFLIB_Hyst_SF_FLT/2
  GFLIB_Hyst_SF_FLT/2 -> Unit Delay/1
  GFLIB_Hyst_SF_FLT/1 -> s32Out/1
  s32In/1 -> GFLIB_Hyst_SF_FLT/1

== system BAMLIB564xL/General Functions/GFLIB_IntegratorTR ==
  note: ---------------------------------------------------------------------------------------------------------------------------------------------------------------------------------------------------
  s32In : Inport
  GFLIB_IntegratorTR_SF_FLT : S-Function  FunctionName=GFLIB_IntegratorTR_SF_FLT  Parameters=s32C1  SFunctionDeploymentMode=off  EnableBusSupport=off
  Unit Delay : UnitDelay  SampleTime=-1
  Unit Delay1 : UnitDelay  SampleTime=-1
  copyright : Subsystem
      mask Display: text(10,90,'FILE:');text(10,75,'DESRIPTION:')text(10,60,'COPYRIGHT:')text(10,45,'VERSION:')text(10,30,'DATE:')text(10,15,'AUTHOR:')
  copyright2 : Subsystem
      mask Display: text(10,90,'GFLIB_IntegratorTR_BAM_FLT.mdl');text(10,75,'Discrete integrator transformed from linear model using Billinear (trapezoidal) transformation.');text(10,60,'Freescale')text(10,45,'0.1');text(10,30,'29-Sep-2010');text(10,15,'');
  logo : Subsystem
      mask Display: image(imread('logo.jpg'))
  s32Out : Outport
  wires:
  Unit Delay1/1 -> GFLIB_IntegratorTR_SF_FLT/2
  Unit Delay/1 -> GFLIB_IntegratorTR_SF_FLT/3
  GFLIB_IntegratorTR_SF_FLT/2 -> Unit Delay1/1
  GFLIB_IntegratorTR_SF_FLT/3 -> Unit Delay/1
  GFLIB_IntegratorTR_SF_FLT/1 -> s32Out/1
  s32In/1 -> GFLIB_IntegratorTR_SF_FLT/1

== system BAMLIB564xL/General Functions/GFLIB_Limit ==
  note: ---------------------------------------------------------------------------------------------------------------------------------------------------------------------------------------------------
  s32In : Inport
  GFLIB_Limit_SF_FLT : S-Function  FunctionName=GFLIB_Limit_SF_FLT  Parameters=s32UpperLimit,s32LowerLim  SFunctionDeploymentMode=off  EnableBusSupport=off
  copyright : Subsystem
      mask Display: text(10,90,'FILE:');text(10,75,'DESRIPTION:')text(10,60,'COPYRIGHT:')text(10,45,'VERSION:')text(10,30,'DATE:')text(10,15,'AUTHOR:')
  copyright2 : Subsystem
      mask Display: text(10,90,'GFLIB_Limit_BAM_FLT.mdl');text(10,75,'Limit function');text(10,60,'Freescale')text(10,45,'0.1');text(10,30,'29-Sep-2010');text(10,15,'');
  logo : Subsystem
      mask Display: image(imread('logo.jpg'))
  s32Out : Outport
  wires:
  GFLIB_Limit_SF_FLT/1 -> s32Out/1
  s32In/1 -> GFLIB_Limit_SF_FLT/1

== system BAMLIB564xL/General Functions/GFLIB_LowerLimit ==
  note: ---------------------------------------------------------------------------------------------------------------------------------------------------------------------------------------------------
  s32In : Inport
  GFLIB_LowerLimit_SF_FLT : S-Function  FunctionName=GFLIB_LowerLimit_SF_FLT  Parameters=s32LowerLim  SFunctionDeploymentMode=off  EnableBusSupport=off
  copyright : Subsystem
      mask Display: text(10,90,'FILE:');text(10,75,'DESRIPTION:')text(10,60,'COPYRIGHT:')text(10,45,'VERSION:')text(10,30,'DATE:')text(10,15,'AUTHOR:')
  copyright2 : Subsystem
      mask Display: text(10,90,'GFLIB_LowerLimit_BAM_FLT.mdl');text(10,75,'Lower limit function');text(10,60,'Freescale')text(10,45,'0.1');text(10,30,'29-Sep-2010');text(10,15,'');
  logo : Subsystem
      mask Display: image(imread('logo.jpg'))
  s32Out : Outport
  wires:
  GFLIB_LowerLimit_SF_FLT/1 -> s32Out/1
  s32In/1 -> GFLIB_LowerLimit_SF_FLT/1

== system BAMLIB564xL/General Functions/GFLIB_Lut1D ==
  note: ---------------------------------------------------------------------------------------------------------------------------------------------------------------------------------------------------
  s32In : Inport
  GFLIB_Lut1D_SF_FLT : S-Function  FunctionName=GFLIB_Lut1D_SF_FLT  Parameters=s32ShamOffset,ps32Table,s32MidIdx  SFunctionDeploymentMode=off  EnableBusSupport=off
  copyright : Subsystem
      mask Display: text(10,90,'FILE:');text(10,75,'DESRIPTION:')text(10,60,'COPYRIGHT:')text(10,45,'VERSION:')text(10,30,'DATE:')text(10,15,'AUTHOR:')
  copyright2 : Subsystem
      mask Display: text(10,90,'GFLIB_Lut1D_BAM_FLT.mdl');text(10,75,'One dimensional Look-up table function');text(10,60,'Freescale')text(10,45,'0.1');text(10,30,'03-Jan-2011');text(10,15,'');
  logo : Subsystem
      mask Display: image(imread('logo.jpg'))
  s32Out : Outport
  wires:
  GFLIB_Lut1D_SF_FLT/1 -> s32Out/1
  s32In/1 -> GFLIB_Lut1D_SF_FLT/1

== system BAMLIB564xL/General Functions/GFLIB_Lut2D ==
  note: ---------------------------------------------------------------------------------------------------------------------------------------------------------------------------------------------------
  s32In1 : Inport
  s32In2 : Inport  Port=2
  GFLIB_Lut2D_SF_FLT : S-Function  FunctionName=GFLIB_Lut2D_SF_FLT  Parameters=s32ShamOffset1,s32ShamOffset2,ps32Table,s32MidId  SFunctionDeploymentMode=off  EnableBusSupport=off
  copyright : Subsystem
      mask Display: text(10,90,'FILE:');text(10,75,'DESRIPTION:')text(10,60,'COPYRIGHT:')text(10,45,'VERSION:')text(10,30,'DATE:')text(10,15,'AUTHOR:')
  copyright2 : Subsystem
      mask Display: text(10,90,'GFLIB_Lut2D_BAM_FLT.mdl');text(10,75,'Two dimensional Look-up table function');text(10,60,'Freescale')text(10,45,'0.1');text(10,30,'03-Jan-2011');text(10,15,'');
  logo : Subsystem
      mask Display: image(imread('logo.jpg'))
  s32Out : Outport
  wires:
  GFLIB_Lut2D_SF_FLT/1 -> s32Out/1
  s32In2/1 -> GFLIB_Lut2D_SF_FLT/2
  s32In1/1 -> GFLIB_Lut2D_SF_FLT/1

== system BAMLIB564xL/General Functions/GFLIB_Ramp ==
  note: ---------------------------------------------------------------------------------------------------------------------------------------------------------------------------------------------------
  s32In : Inport
  GFLIB_Ramp_SF_FLT : S-Function  FunctionName=GFLIB_Ramp_SF_FLT  Parameters=s32RampUp,s32RampDown  SFunctionDeploymentMode=off  EnableBusSupport=off
  Unit Delay : UnitDelay  SampleTime=-1
  copyright : Subsystem
      mask Display: text(10,90,'FILE:');text(10,75,'DESRIPTION:')text(10,60,'COPYRIGHT:')text(10,45,'VERSION:')text(10,30,'DATE:')text(10,15,'AUTHOR:')
  copyright2 : Subsystem
      mask Display: text(10,90,'GFLIB_Ramp_BAM_FLT.mdl');text(10,75,'Rate of change limiter - Ramp function.');text(10,60,'Freescale')text(10,45,'0.1');text(10,30,'29-Sep-2010');text(10,15,'');
  logo : Subsystem
      mask Display: image(imread('logo.jpg'))
  s32Out : Outport
  wires:
  Unit Delay/1 -> GFLIB_Ramp_SF_FLT/2
  GFLIB_Ramp_SF_FLT/2 -> Unit Delay/1
  GFLIB_Ramp_SF_FLT/1 -> s32Out/1
  s32In/1 -> GFLIB_Ramp_SF_FLT/1

== system BAMLIB564xL/General Functions/GFLIB_Sign ==
  note: ---------------------------------------------------------------------------------------------------------------------------------------------------------------------------------------------------
  s32In : Inport
  GFLIB_Sign_SF_FLT : S-Function  FunctionName=GFLIB_Sign_SF_FLT  SFunctionDeploymentMode=off  EnableBusSupport=off
  copyright : Subsystem
      mask Display: text(10,90,'FILE:');text(10,75,'DESRIPTION:')text(10,60,'COPYRIGHT:')text(10,45,'VERSION:')text(10,30,'DATE:')text(10,15,'AUTHOR:')
  copyright2 : Subsystem
      mask Display: text(10,90,'GFLIB_Sign_BAM_FLT.mdl');text(10,75,'Sign function');text(10,60,'Freescale')text(10,45,'0.1');text(10,30,'29-Sep-2010');text(10,15,'');
  logo : Subsystem
      mask Display: image(imread('logo.jpg'))
  s32Out : Outport
  wires:
  GFLIB_Sign_SF_FLT/1 -> s32Out/1
  s32In/1 -> GFLIB_Sign_SF_FLT/1
